simulink model "lab5_rlc_block"  (R2024a)
settings: Solver=VariableStepAuto  StartTime=0.0  StopTime=10.0  RelTol=1e-3
settings Model: Creator=Admin  LastModifiedBy=Admin

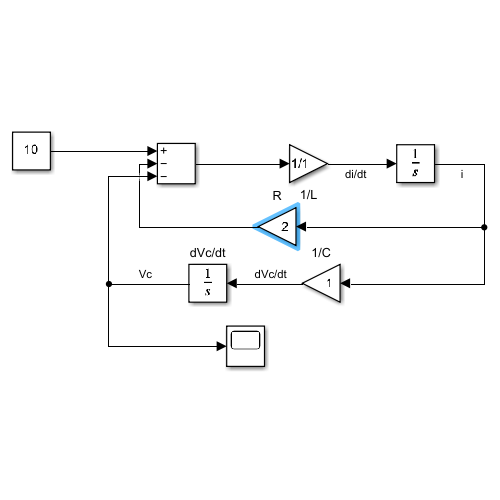
[thumbnail: Simulink's stored preview of the top-level diagram]
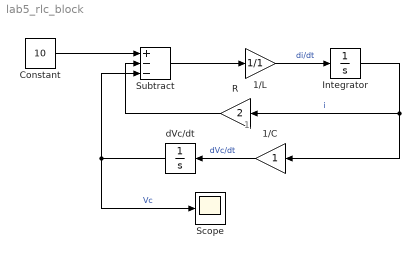
== system lab5_rlc_block ==
  note: 1
  1/C : Gain
  1/L : Gain  Gain=1/1
  Constant : Constant  Value=10
  Integrator : Integrator
  R : Gain  Gain=2
  Scope : Scope
  Subtract : Sum  Inputs=+--
  dVc/dt : Integrator
  wires:
  1/L/1 -> Integrator/1  "di/dt"
  Integrator/1 -> 1/C/1, R/1  "i"
  1/C/1 -> dVc/dt/1  "dVc/dt"
  Constant/1 -> Subtract/1
  R/1 -> Subtract/2
  dVc/dt/1 -> Scope/1, Subtract/3  "Vc"
  Subtract/1 -> 1/L/1
